simulink model "ljsbirkhoff"  (Simulink 4.00)
settings: Solver=ode45  SolverMode=SingleTasking  StartTime=60  StopTime=240  RelTol=1e-3  AbsTol=1e-6
libraries: simulink3 x1
settings Model: LastModifiedBy=LJS  LimitDataPoints=off

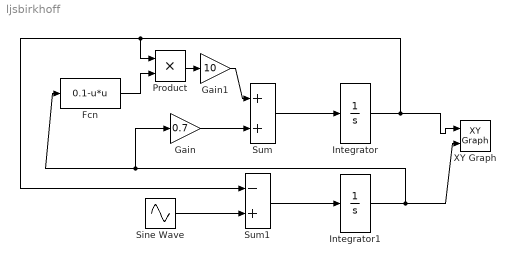
== system ljsbirkhoff ==
  Fcn : Fcn  Expr=0.1-u*u
  Gain : Gain  Gain=0.7  Multiplication=Element-wise(K.*u)  SaturateOnIntegerOverflow=on
  Gain1 : Gain  Gain=10  Multiplication=Element-wise(K.*u)  SaturateOnIntegerOverflow=on
  Integrator : Integrator  ExternalReset=none  InitialConditionSource=internal  InitialCondition=1  LimitOutput=off  UpperSaturationLimit=inf  LowerSaturationLimit=-inf  ShowSaturationPort=off  ShowStatePort=off  AbsoluteTolerance=auto
  Integrator1 : Integrator  ExternalReset=none  InitialConditionSource=internal  InitialCondition=1  LimitOutput=off  UpperSaturationLimit=inf  LowerSaturationLimit=-inf  ShowSaturationPort=off  ShowStatePort=off  AbsoluteTolerance=auto
  Product : Product  Inputs=2  Multiplication=Element-wise(.*)  SaturateOnIntegerOverflow=on
  Sine Wave : Sin  SineType=Time-based  Amplitude=0.25  Bias=0  Frequency=pi/2  Phase=0  Samples=10  SampleTime=0  Offset=0
  Sum : Sum  Inputs=++  SaturateOnIntegerOverflow=on
  Sum1 : Sum  Inputs=-+  SaturateOnIntegerOverflow=on
  XY Graph : simulink3/Sinks/XY Graph  xmin=-1  xmax=1  ymin=-1  ymax=1  st=0.01
  wires:
  Sum/1 -> Integrator/1
  Sum1/1 -> Integrator1/1
  Gain/1 -> Sum/2
  Integrator1/1 -> XY Graph/2, Gain/1, Fcn/1
  Fcn/1 -> Product/2
  Integrator/1 -> XY Graph/1, Product/1, Sum1/1
  Product/1 -> Gain1/1
  Gain1/1 -> Sum/1
  Sine Wave/1 -> Sum1/2
